simulink model "flyback_imc"  (R2021b)
settings: Solver=FixedStepDiscrete  StartTime=0.0  StopTime=100e-3  RelTol=1e-3
Description:
  | Symmetric FIR Filter
  | This example shows how to use HDL Coder(TM) to check, generate,
  | and verify HDL for a fixed-point symmetric FIR filter.
settings Model: DataTypeOverride=Off  Creator=The MathWorks, Inc.  LastModifiedBy=Marco Milanesi
settings SolverCC: AlgebraicLoopSolver=TrustRegion  AutoInsertRateTranBlk=on
settings DataIOCC: LimitDataPoints=on  SaveFormat=Array  SaveOutput=off  SignalLogging=off  SaveTime=off  ReturnWorkspaceOutputs=off  SignalLoggingName=logsOut
settings OptimizationCC: BlockReduction=off  BooleanDataType=off  ConditionallyExecuteInputs=off  DefaultParameterBehavior=Inlined  InheritOutputTypeSmallerThanSingle=on  InlineInvariantSignals=on  ExpressionDepthLimit=2147483647  InitFltsAndDblsToZero=on  LifeSpan=inf  BufferReusableBoundary=off
settings DebuggingCC: AlgebraicLoopMsg=error  SaveWithParameterizedLinksMsg=none  UnderspecifiedInitializationDetection=Classic  MergeDetectMultiDrivingBlocksExec=none  CheckExecutionContextPreStartOutputMsg=on  SignalResolutionControl=TryResolveAllWithWarning  MultiTaskDSMMsg=warning  MultiTaskCondExecSysMsg=none  SingleTaskRateTransMsg=error  IntegerOverflowMsg=none  ParameterPrecisionLossMsg=none  FcnCallInpInsideContextMsg=warning  BusObjectLabelMismatch=none  StateNameClashWarn=warning  SFUnexpectedBacktrackingDiag=warning  SFNoUnconditionalDefaultTransitionDiag=warning  SFExecutionAtInitializationDiag=none  SFMachineParentedDataDiag=warning  IntegerSaturationMsg=none  ArithmeticOperatorsInVariantConditions=warning
settings HardwareCC: ProdBitPerPointer=32  ProdBitPerSizeT=32  ProdBitPerPtrDiffT=32  ProdLargestAtomicFloat=None  ProdIntDivRoundTo=Undefined  ProdEndianess=Unspecified  ProdWordSize=32  ProdHWDeviceType=ASIC/FPGA  TargetUnknown=on  ProdEqTarget=off
settings ModelReferenceCC: PropagateSignalLabelsOutOfModel=off
settings SFSimCC: SimUseLocalCustomCode=off  CustomCodeUndefinedFunction=UseInterfaceOnly
settings RTWCC: RTWUseLocalCustomCode=off
settings CodeAppCC: StateflowObjectComments=on
settings GRTTargetCC: TargetFcnLib=ansi_tfl_tmw.mat  TargetLangStandard=C89/C90 (ANSI)  CombineOutputUpdateFcns=off  GRTInterface=on
settings ConfigComp: CovMetricSettings=dw  CovSaveCumulativeToWorkspaceVar=on  CovSaveSingleToWorkspaceVar=on  CovExternalEMLEnable=off

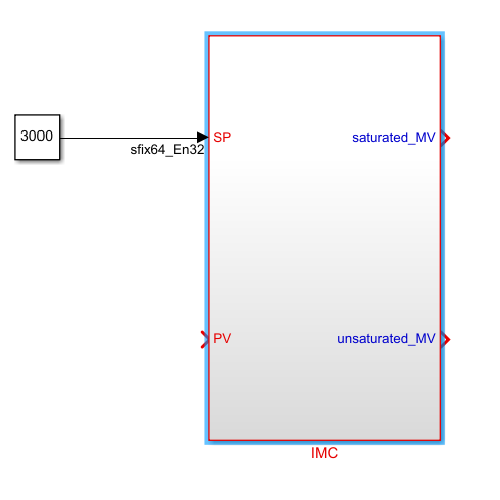
[thumbnail: Simulink's stored preview of the top-level diagram]
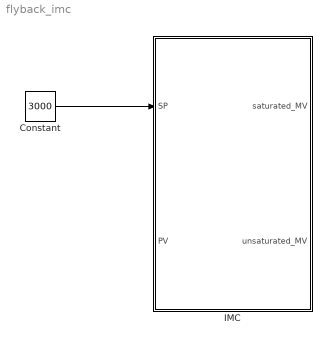
== system flyback_imc ==
  Constant : Constant  Value=3000
  IMC : Subsystem
  wires:
  Constant/1 -> IMC/1(SP)

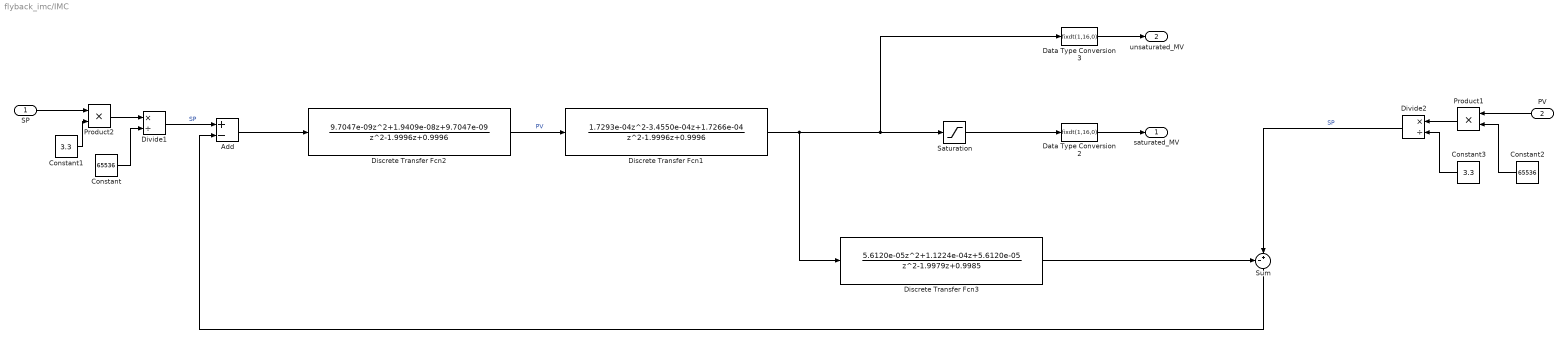
== system flyback_imc/IMC ==
  SP : Inport  OutDataTypeStr=fixdt(1,64,32)  SampleTime=80e-9
  PV : Inport  Port=2  OutDataTypeStr=fixdt(1,64,32)  SampleTime=80e-9
  Add : Sum  Inputs=+-
  Constant : Constant  Value=65536  OutDataTypeStr=fixdt(1,64,32)
  Constant1 : Constant  Value=3.3  OutDataTypeStr=fixdt(1,64,32)
  Constant2 : Constant  Value=65536  OutDataTypeStr=fixdt(1,64,32)
  Constant3 : Constant  Value=3.3  OutDataTypeStr=fixdt(1,64,32)
  Data Type Conversion2 : DataTypeConversion  OutDataTypeStr=fixdt(1,16,0)
  Data Type Conversion3 : DataTypeConversion  OutDataTypeStr=fixdt(1,16,0)
  Discrete Transfer Fcn1 : DiscreteTransferFcn  Numerator=[1.7293e-04 -3.4550e-04 1.7266e-04]  Denominator=[1 -1.9996 0.9996]  SampleTime=0.00001  NumCoefDataTypeStr=fixdt(1,64,32)  DenCoefDataTypeStr=fixdt(1,64,32)  NumProductDataTypeStr=fixdt(1,64,32)  DenProductDataTypeStr=fixdt(1,64,32)  NumAccumDataTypeStr=fixdt(1,64,32)  DenAccumDataTypeStr=fixdt(1,64,32)  OutDataTypeStr=fixdt(1,64,32)
  Discrete Transfer Fcn2 : DiscreteTransferFcn  Numerator=[9.7047e-09 1.9409e-08 9.7047e-09]  Denominator=[1 -1.9996 0.9996]  SampleTime=0.00001  NumCoefDataTypeStr=fixdt(1,64,32)  DenCoefDataTypeStr=fixdt(1,64,32)  NumProductDataTypeStr=fixdt(1,64,32)  DenProductDataTypeStr=fixdt(1,64,32)  NumAccumDataTypeStr=fixdt(1,64,32)  DenAccumDataTypeStr=fixdt(1,64,32)  OutDataTypeStr=fixdt(1,64,32)
  Discrete Transfer Fcn3 : DiscreteTransferFcn  Numerator=[5.6120e-05 1.1224e-04 5.6120e-05]  Denominator=[1 -1.9979 0.9985]  SampleTime=0.00001  NumCoefDataTypeStr=fixdt(1,64,32)  DenCoefDataTypeStr=fixdt(1,64,32)  NumProductDataTypeStr=fixdt(1,64,32)  DenProductDataTypeStr=fixdt(1,64,32)  NumAccumDataTypeStr=fixdt(1,64,32)  DenAccumDataTypeStr=fixdt(1,64,32)  OutDataTypeStr=fixdt(1,64,32)
  Divide1 : Product  Inputs=*/  RndMeth=Zero  SaturateOnIntegerOverflow=on  LockScale=on
  Divide2 : Product  Inputs=*/  RndMeth=Zero  SaturateOnIntegerOverflow=on  LockScale=on
  Product1 : Product  OutDataTypeStr=fixdt(1,64,32)
  Product2 : Product  OutDataTypeStr=fixdt(1,64,32)
  Saturation : Saturate  UpperLimit=255  LowerLimit=0  OutDataTypeStr=fixdt(1,16,0)
  Sum : Sum  Inputs=-+|
  saturated_MV : Outport  OutDataTypeStr=fixdt(1,16,0)  SampleTime=80e-9  VectorParamsAs1DForOutWhenUnconnected=off
  unsaturated_MV : Outport  Port=2  OutDataTypeStr=fixdt(1,16,0)  SampleTime=80e-9  VectorParamsAs1DForOutWhenUnconnected=off
  wires:
  Data Type Conversion2/1 -> saturated_MV/1
  Saturation/1 -> Data Type Conversion2/1
  Discrete Transfer Fcn1/1 -> Discrete Transfer Fcn3/1, Saturation/1, Data Type Conversion3/1
  Data Type Conversion3/1 -> unsaturated_MV/1
  Add/1 -> Discrete Transfer Fcn2/1
  Discrete Transfer Fcn2/1 -> Discrete Transfer Fcn1/1  "PV"
  Discrete Transfer Fcn3/1 -> Sum/1
  Sum/1 -> Add/2
  SP/1 -> Product2/1
  Product2/1 -> Divide1/1
  Constant/1 -> Divide1/2
  Constant1/1 -> Product2/2
  Divide1/1 -> Add/1  "SP"
  Product1/1 -> Divide2/1
  PV/1 -> Product1/1
  Divide2/1 -> Sum/2  "SP"
  Constant3/1 -> Divide2/2
  Constant2/1 -> Product1/2
